simulink model "FOC_FPGA"  (R2020a)
settings: Solver=FixedStepDiscrete  StartTime=0.0  StopTime=1  FixedStep=2e-6  MaxStep=1e-4  RelTol=1e-3
values from neighbouring files (symbols this model uses):
  Ld = 0.008    [Thong_so_dong_co_FOC.m]
  Lq = 0.008    [Thong_so_dong_co_FOC.m]
  Omega = exp(-wc*Tp_SMO)    [Thong_so_dong_co_FOC.m]
  T_pulse = 5*10^(-5)    (= 5e-05)    [Thong_so_dong_co_FOC.m]
  Ts_idq = 1*10^(-4)    (= 0.0001)    [Thong_so_dong_co_FOC.m]
  Wc = exp(-500*Tp_SMO)    [Thong_so_dong_co_FOC.m]
  zp = 4    [Thong_so_dong_co_FOC.m]
undefined symbols (not defined in the file or in its folder): Inventor, PMSM
libraries: powerlib x11, modelsimlib x6, simulink x1
settings Model: Creator=ADMIN  LastModifiedBy=ADMIN
settings SolverCC: ZeroCrossAlgorithm=Adaptive
settings DebuggingCC: IgnoredZcDiagnostic=none

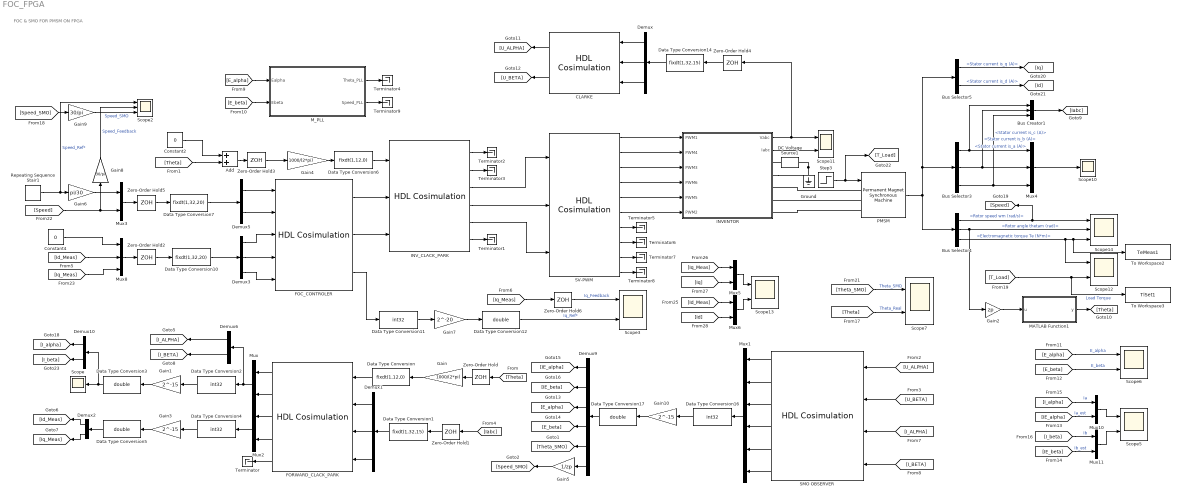
== system FOC_FPGA ==
  note: FOC & SMO FOR PMSM ON FPGA
  Add : Sum
  Bus Creator1 : BusCreator  Inputs=3
  Bus Selector3 : BusSelector  OutputSignals=Stator current is_a (A),Stator current is_b (A),Stator current is_c (A)
  Bus Selector4 : BusSelector  OutputSignals=Rotor speed wm (rad/s),Rotor angle thetam (rad),Electromagnetic torque Te (N*m)
  Bus Selector5 : BusSelector  OutputSignals=Stator current is_q (A),Stator current is_d (A)
  CLARKE : modelsimlib/HDL Cosimulation  PortPaths=/clarke/UA;/clarke/UB;/clarke/UC;/clarke/U_ALPHA;/clarke/U_BETA  PortModes=[1 1 1 2 2 ]  PortTimes=[-1,-1,-1,2e-6,2e-6]  PortSigns=[-1 -1 -1 -1 -1 ]  PortFracLengths=[0,0,0,0,0]  CommLocal=on  CommSharedMemory=on  CommPortNumber=4449  CommShowInfo=on  ClockPaths=/clarke/CLK  ClockModes=[2 ]  ClockTimes=[2e-8]  TclPreSimCommand="puts \"Running Simulink Cosimulation block.\""  TclPostSimCommand="puts \"done\""  TimingMode=s  TimingScaleFactor=1  idxCellArray={'UNUSED_VAR'}  CosimBypass=Full Simulation  AllowDirectFeedthrough=on  ProductName=EDA Simulator Link MQ  RunAutoTimescale=off  HdlClocks=0  PreRunTime=0  PreRunTimeUnit=ns
      settings: SourceProductBaseCode=ES
  Constant2 : Constant  Value=0
  Constant4 : Constant  Value=0
  DC Voltage Source1 : powerlib/Electrical Sources/DC Voltage Source  Amplitude=100  Measurements=None
  Data Type Conversion : DataTypeConversion  OutDataTypeStr=fixdt(1,12,0)
  Data Type Conversion1 : DataTypeConversion  OutDataTypeStr=fixdt(1,32,15)
  Data Type Conversion10 : DataTypeConversion  OutDataTypeStr=fixdt(1,32,20)
  Data Type Conversion{2,4,11,16} (4 alike) : DataTypeConversion  OutDataTypeStr=int32
  Data Type Conversion{3,5,12,17} (4 alike) : DataTypeConversion  OutDataTypeStr=double
  Data Type Conversion14 : DataTypeConversion  OutDataTypeStr=fixdt(1,32,15)
  Data Type Conversion6 : DataTypeConversion  OutDataTypeStr=fixdt(1,12,0)
  Data Type Conversion7 : DataTypeConversion  OutDataTypeStr=fixdt(1,32,20)
  Demux : Demux  Outputs=3
  Demux1 : Demux  Outputs=3
  Demux{2,5..6,10} (4 alike) : Demux  Outputs=2
  Demux3 : Demux  Outputs=3
  Demux9 : Demux  Outputs=6
  FOC_CONTROLER : modelsimlib/HDL Cosimulation  PortPaths=/foc_control/W_REF;/foc_control/W;/foc_control/I_DR;/foc_control/I_D;/foc_control/I_Q;/foc_control/U_D;/foc_control/U_Q;/foc_control/I_QR  PortModes=[1 1 1 1 1 2 2 2 ]  PortTimes=[-1,-1,-1,-1,-1,2e-6,2e-6,2e-6]  PortSigns=[-1 -1 -1 -1 -1 -1 -1 -1 ]  PortFracLengths=[0,0,0,0,0,0,0,0]  CommLocal=on  CommSharedMemory=on  CommPortNumber=4449  CommShowInfo=on  ClockPaths=/foc_control/CLK;/foc_control/CLK_200N  ClockModes=[2 2 ]  ClockTimes=[2e-8,2e-7]  TclPreSimCommand="puts \"Running Simulink Cosimulation block.\""  TclPostSimCommand="puts \"done\""  TimingMode=s  TimingScaleFactor=1  idxCellArray={'UNUSED_VAR'}  CosimBypass=Full Simulation  AllowDirectFeedthrough=on  ProductName=EDA Simulator Link MQ  RunAutoTimescale=off  HdlClocks=0  PreRunTime=0  PreRunTimeUnit=ns
      settings: SourceProductBaseCode=ES
  FORWARD_CLACK_PARK : modelsimlib/HDL Cosimulation  PortPaths=/forward_clack_park/ADDRESS;/forward_clack_park/IA;/forward_clack_park/IB;/forward_clack_park/IC;/forward_clack_park/I_ALPHA;/forward_clack_park/I_BETA;/forward_clack_park/I_D;/forward_clack_park/I_Q;/forward_clack_park/DONE  PortModes=[1 1 1 1 2 2 2 2 2 ]  PortTimes=[-1,-1,-1,-1,2e-6,2e-6,2e-6,2e-6,2e-6]  PortSigns=[-1 -1 -1 -1 -1 -1 -1 -1 -1 ]  PortFracLengths=[0,0,0,0,0,0,0,0,0]  CommLocal=on  CommSharedMemory=on  CommPortNumber=4449  CommShowInfo=on  ClockPaths=/forward_clack_park/CLK  ClockModes=[2 ]  ClockTimes=[2e-8]  TclPreSimCommand="puts \"Running Simulink Cosimulation block.\""  TclPostSimCommand="puts \"done\""  TimingMode=s  TimingScaleFactor=1  idxCellArray={'UNUSED_VAR'}  CosimBypass=Full Simulation  AllowDirectFeedthrough=on  ProductName=EDA Simulator Link MQ  RunAutoTimescale=off  HdlClocks=0  PreRunTime=0  PreRunTimeUnit=ns
      settings: SourceProductBaseCode=ES
  Gain : Gain  Gain=1000/(2*pi)
  Gain1 : Gain  Gain=2^-15
  Gain10 : Gain  Gain=2^-15
  Gain2 : Gain  Gain=zp
  Gain3 : Gain  Gain=2^-15
  Gain4 : Gain  Gain=1000/(2*pi)
  Gain5 : Gain  Gain=1/zp
  Gain6 : Gain  Gain=pi/30
  Gain7 : Gain  Gain=2^-20
  Gain8 : Gain  Gain=30/pi
  Gain9 : Gain  Gain=30/pi
  Ground : powerlib/Elements/Ground  LConnTagsString=a
  INVENTOR : Subsystem  AncestorBlock=PMSM/Inventor
  INV_CLACK_PARK : modelsimlib/HDL Cosimulation  PortPaths=/inverse_clack_park/ADDRESS;/inverse_clack_park/U_D;/inverse_clack_park/U_Q;/inverse_clack_park/U_ALPHA;/inverse_clack_park/U_BETA;/inverse_clack_park/VREFA;/inverse_clack_park/VREFB;/inverse_clack_park/VREFC;/inverse_clack_park/DONE  PortModes=[1 1 1 2 2 2 2 2 2 ]  PortTimes=[-1,-1,-1,2e-6,2e-6,2e-6,2e-6,2e-6,2e-6]  PortSigns=[-1 -1 -1 -1 -1 -1 -1 -1 -1 ]  PortFracLengths=[0,0,0,0,0,0,0,0,0]  CommLocal=on  CommSharedMemory=on  CommPortNumber=4449  CommShowInfo=on  ClockPaths=/inverse_clack_park/CLK  ClockModes=[2 ]  ClockTimes=[2e-8]  TclPreSimCommand="puts \"Running Simulink Cosimulation block.\""  TclPostSimCommand="puts \"done\""  TimingMode=s  TimingScaleFactor=1  idxCellArray={'UNUSED_VAR'}  CosimBypass=Full Simulation  AllowDirectFeedthrough=on  ProductName=EDA Simulator Link MQ  RunAutoTimescale=off  HdlClocks=0  PreRunTime=0  PreRunTimeUnit=ns
      settings: SourceProductBaseCode=ES
  MATLAB Function1 : MATLAB Function  TreatAsAtomicUnit=on
  M_PLL : Subsystem
  Mux{,2..3,5..6,10..11} (7 alike) : Mux  Inputs=2
  Mux1 : Mux  Inputs=6
  Mux4 : Mux  Inputs=3
  Mux8 : Mux  Inputs=3
  PMSM : powerlib/Machines/Permanent Magnet Synchronous Machine  NbPhases=3  FluxDistribution=Sinusoidal  RotorType=Salient-pole  MechanicalLoad=Torque Tm  PresetModel=No  ShowDetailedParameters=on  MeasurementBus=off  Resistance=3.2  Inductance=8.5e-3  dqInductances=[Ld Lq]  La=0.008  MachineConstant=Flux linkage established by magnets (V.s)  Flux=0.0471405  VoltageCst=34.2014  TorqueCst=0.28284  Flat=120  Mechanical=[1.4e-05 4.5e-06 4]  PolePairs=2  InitialConditions=[0,0, 0,0]  InitialConditions5ph=[0 0 0 0 0 0]  RefAngle=Aligned with phase A axis (original Park)  IterativeDiscreteModel=Trapezoidal non iterative  TsBlock=-1  TsPowergui=0
  Repeating Sequence Stair1 : simulink/Sources/Repeating Sequence Stair  OutValues=[300 600 900 -600 -300 ].'  tsamp=0.2  OutMin=[]  OutMax=[]  OutDataTypeStr=double  OutputDataTypeScalingMode=double  OutDataType=fixdt(0,8)  ConRadixGroup=Best Precision: Vector-wise  OutScaling=2^-12
  SMO OBSERVER : modelsimlib/HDL Cosimulation  PortPaths=/smo_observer/U_ALPHA;/smo_observer/U_BETA;/smo_observer/I_ALPHA;/smo_observer/I_BETA;/smo_observer/IE_ALPHA;/smo_observer/IE_BETA;/smo_observer/E_ALPHA;/smo_observer/E_BETA;/smo_observer/THETA;/smo_observer/SPEED  PortModes=[1 1 1 1 2 2 2 2 2 2 ]  PortTimes=[-1,-1,-1,-1,2e-6,2e-6,2e-6,2e-6,2e-6,2e-6]  PortSigns=[-1 -1 -1 -1 -1 -1 -1 -1 -1 -1 ]  PortFracLengths=[0,0,0,0,0,0,0,0,0,0]  CommLocal=on  CommSharedMemory=on  CommPortNumber=4449  CommShowInfo=on  ClockPaths=/smo_observer/CLK;/smo_observer/CLK_80N  ClockModes=[2 2 ]  ClockTimes=[2e-8,8e-8]  TclPreSimCommand="puts \"Running Simulink Cosimulation block.\""  TclPostSimCommand="puts \"done\""  TimingMode=s  TimingScaleFactor=1  idxCellArray={'UNUSED_VAR'}  CosimBypass=Full Simulation  AllowDirectFeedthrough=on  ProductName=EDA Simulator Link MQ  RunAutoTimescale=off  HdlClocks=0  PreRunTime=0  PreRunTimeUnit=ns
      settings: SourceProductBaseCode=ES
  SV-PWM : modelsimlib/HDL Cosimulation  PortPaths=/svpwm/VREF1;/svpwm/VREF2;/svpwm/VREF3;/svpwm/PWM1;/svpwm/PWM2;/svpwm/PWM3;/svpwm/PWM4;/svpwm/PWM5;/svpwm/PWM6;/svpwm/CMPR1;/svpwm/CMPR2;/svpwm/CMPR3;/svpwm/Q  PortModes=[1 1 1 2 2 2 2 2 2 2 2 2 2 ]  PortTimes=[-1,-1,-1,2e-6,2e-6,2e-6,2e-6,2e-6,2e-6,1,1,1,1]  PortSigns=[-1 -1 -1 -1 -1 -1 -1 -1 -1 -1 -1 -1 -1 ]  PortFracLengths=[0,0,0,0,0,0,0,0,0,0,0,0,0]  CommLocal=on  CommSharedMemory=on  CommPortNumber=4449  CommShowInfo=on  ClockPaths=/svpwm/CLK;/svpwm/CLK_200N  ClockModes=[2 2 ]  ClockTimes=[2e-8,2e-7]  TclPreSimCommand="puts \"Running Simulink Cosimulation block.\""  TclPostSimCommand="puts \"done\""  TimingMode=s  TimingScaleFactor=1  idxCellArray={'UNUSED_VAR'}  CosimBypass=Full Simulation  AllowDirectFeedthrough=on  ProductName=EDA Simulator Link MQ  RunAutoTimescale=off  HdlClocks=0  PreRunTime=0  PreRunTimeUnit=ns
      settings: SourceProductBaseCode=ES
  Scope : Scope
  Scope10 : Scope
  Scope{3,5..7,11..13} (7 alike) : Scope  NumInputPorts=2
  Scope14 : Scope  NumInputPorts=3
  Scope2 : Scope  NumInputPorts=3
  Step3 : Step  Time=0.15  Before=0.2  After=0.3  SampleTime=0
  Terminator{,1..9} (10 alike) : Terminator
  To Workspace2 : ToWorkspace  VariableName=TeMeas1  SampleTime=-1
  To Workspace3 : ToWorkspace  VariableName=TlSet1  SampleTime=-1
  Zero-Order Hold{,1..5} (6 alike) : ZeroOrderHold  SampleTime=2e-6
  Zero-Order Hold6 : ZeroOrderHold  SampleTime=Ts_idq
  wires:
  [Iq] -> Mux5/2
  Bus Creator1/1 -> [Iabc]
  [T_Load] -> To Workspace3/1, Scope12/2  "Load Torque"
  Mux6/1 -> Scope13/2
  Bus Selector3/1 -> Bus Creator1/1, Mux4/1  "<Stator current is_a (A)>"
  [Iq_Meas] -> Mux5/1
  INVENTOR/2("Iabc ") -> Scope11/2
  Mux4/1 -> Scope10/1
  PMSM/1 -> Bus Selector4/1, Bus Selector5/1, Bus Selector3/1
  Bus Selector3/3 -> Bus Creator1/3, Mux4/3  "<Stator current is_c (A)>"
  [Id] -> Mux6/2
  Mux5/1 -> Scope13/1
  Bus Selector4/1 -> Scope14/1, [Speed]  "<Rotor speed wm (rad/s)>"
  Step3/1 -> PMSM/1, [T_Load]
  Bus Selector5/1 -> [Iq]  "<Stator current is_q (A)>"
  MATLAB Function1/1(y) -> [Theta]
  Bus Selector4/2 -> Scope14/2, Gain2/1  "<Rotor angle thetam (rad)>"
  Gain2/1 -> MATLAB Function1/1(u)
  [Id_Meas] -> Mux6/1
  Bus Selector3/2 -> Bus Creator1/2, Mux4/2  "<Stator current is_b (A)>"
  Bus Selector4/3 -> Scope12/1, To Workspace2/1, Scope14/3  "<Electromagnetic torque Te (N*m)>"
  Bus Selector5/2 -> [Id]  "<Stator current is_d (A)>"
  [Theta] -> Zero-Order Hold/1
  Zero-Order Hold/1 -> Gain/1
  Gain/1 -> Data Type Conversion/1
  Data Type Conversion/1 -> FORWARD_CLACK_PARK/1
  Demux1/3 -> FORWARD_CLACK_PARK/4
  Demux1/2 -> FORWARD_CLACK_PARK/3
  Demux1/1 -> FORWARD_CLACK_PARK/2
  Data Type Conversion1/1 -> Demux1/1
  Zero-Order Hold1/1 -> Data Type Conversion1/1
  [Iabc] -> Zero-Order Hold1/1
  FORWARD_CLACK_PARK/1 -> Mux/1
  FORWARD_CLACK_PARK/2 -> Mux/2
  Mux/1 -> Demux6/1, Data Type Conversion2/1
  Data Type Conversion2/1 -> Gain1/1
  Gain1/1 -> Data Type Conversion3/1
  Data Type Conversion3/1 -> Scope/1, Demux10/1
  Gain3/1 -> Data Type Conversion5/1
  Data Type Conversion4/1 -> Gain3/1
  Mux2/1 -> Data Type Conversion4/1
  FORWARD_CLACK_PARK/4 -> Mux2/2
  FORWARD_CLACK_PARK/3 -> Mux2/1
  Data Type Conversion5/1 -> Demux2/1
  Demux2/1 -> [Id_Meas]
  Demux2/2 -> [Iq_Meas]
  Data Type Conversion6/1 -> INV_CLACK_PARK/1
  Gain4/1 -> Data Type Conversion6/1
  Zero-Order Hold3/1 -> Gain4/1
  Add/1 -> Zero-Order Hold3/1
  [Theta] -> Add/2
  Constant2/1 -> Add/1
  Repeating Sequence Stair1/1 -> Gain6/1, Scope2/1  "Speed_Ref*"
  Mux8/1 -> Zero-Order Hold2/1
  Data Type Conversion10/1 -> Demux3/1
  FOC_CONTROLER/1 -> INV_CLACK_PARK/2
  FOC_CONTROLER/2 -> INV_CLACK_PARK/3
  [Speed] -> Gain8/1, Mux3/2
  Demux3/2 -> FOC_CONTROLER/4
  Demux3/3 -> FOC_CONTROLER/5
  Demux3/1 -> FOC_CONTROLER/3
  Constant4/1 -> Mux8/1
  Zero-Order Hold2/1 -> Data Type Conversion10/1
  [Id_Meas] -> Mux8/2
  [Iq_Meas] -> Mux8/3
  Zero-Order Hold5/1 -> Data Type Conversion7/1
  Data Type Conversion7/1 -> Demux5/1
  Demux5/1 -> FOC_CONTROLER/1
  Demux5/2 -> FOC_CONTROLER/2
  Mux3/1 -> Zero-Order Hold5/1
  Gain6/1 -> Mux3/1
  Data Type Conversion11/1 -> Gain7/1
  Gain7/1 -> Data Type Conversion12/1
  FOC_CONTROLER/3 -> Data Type Conversion11/1
  [Iq_Meas] -> Zero-Order Hold6/1
  FORWARD_CLACK_PARK/5 -> Terminator/1
  INV_CLACK_PARK/6 -> Terminator1/1
  INV_CLACK_PARK/5 -> SV-PWM/3
  SV-PWM/7 -> Terminator5/1
  SV-PWM/8 -> Terminator6/1
  SV-PWM/9 -> Terminator7/1
  SV-PWM/10 -> Terminator8/1
  INV_CLACK_PARK/3 -> SV-PWM/1
  SV-PWM/1 -> INVENTOR/1("PWM1 ")
  SV-PWM/2 -> INVENTOR/2("PWM4 ")
  SV-PWM/3 -> INVENTOR/3("PWM3 ")
  SV-PWM/4 -> INVENTOR/4("PWM6 ")
  SV-PWM/5 -> INVENTOR/5("PWM5 ")
  SV-PWM/6 -> INVENTOR/6("PWM2 ")
  Gain8/1 -> Scope2/2  "Speed_Feedback"
  Demux6/1 -> [I_ALPHA]
  Demux6/2 -> [I_BETA]
  Data Type Conversion17/1 -> Demux9/1
  Mux1/1 -> Data Type Conversion16/1
  Data Type Conversion16/1 -> Gain10/1
  Gain10/1 -> Data Type Conversion17/1
  Mux10/1 -> Scope5/1
  Mux11/1 -> Scope5/2
  [IE_alpha] -> Mux10/2  "Ia_est"
  [IE_beta] -> Mux11/2  "Ib_est"
  [I_beta] -> Mux11/1  "Ib"
  [I_alpha] -> Mux10/1  "Ia"
  [E_beta] -> Scope6/2  "E_beta"
  [E_alpha] -> Scope6/1  "E_alpha"
  Demux10/1 -> [I_alpha]
  Demux10/2 -> [I_beta]
  INVENTOR/1("Vabc ") -> Scope11/1, Zero-Order Hold4/1
  Data Type Conversion12/1 -> Scope3/2  "Iq_Ref*"
  Zero-Order Hold6/1 -> Scope3/1  "Iq_Feedback"
  INV_CLACK_PARK/4 -> SV-PWM/2
  Demux/3 -> CLARKE/3
  Demux/2 -> CLARKE/2
  Demux/1 -> CLARKE/1
  [Speed_SMO] -> Gain9/1
  Gain9/1 -> Scope2/3  "Speed_SMO"
  Zero-Order Hold4/1 -> Data Type Conversion14/1
  Data Type Conversion14/1 -> Demux/1
  CLARKE/1 -> [U_ALPHA]
  CLARKE/2 -> [U_BETA]
  [E_alpha] -> M_PLL/1(Ealpha)
  [E_beta] -> M_PLL/2(Ebeta)
  [I_ALPHA] -> SMO OBSERVER/3
  [I_BETA] -> SMO OBSERVER/4
  [U_BETA] -> SMO OBSERVER/2
  [U_ALPHA] -> SMO OBSERVER/1
  SMO OBSERVER/1 -> Mux1/1
  SMO OBSERVER/4 -> Mux1/4
  SMO OBSERVER/5 -> Mux1/5
  SMO OBSERVER/3 -> Mux1/3
  SMO OBSERVER/2 -> Mux1/2
  Demux9/1 -> [IE_alpha]
  Demux9/2 -> [IE_beta]
  Demux9/3 -> [E_alpha]
  Demux9/4 -> [E_beta]
  Demux9/5 -> [Theta_SMO]
  INV_CLACK_PARK/2 -> Terminator3/1
  INV_CLACK_PARK/1 -> Terminator2/1
  SMO OBSERVER/6 -> Mux1/6
  Demux9/6 -> Gain5/1
  [Theta_SMO] -> Scope7/1  "Theta_SMO"
  [Theta] -> Scope7/2  "Theta_Real"
  M_PLL/2(Speed_PLL) -> Terminator9/1
  M_PLL/1(Theta_PLL) -> Terminator4/1
  Gain5/1 -> [Speed_SMO]
  connections:
  INVENTOR/RConn2 -- Ground/LConn1 -- DC Voltage Source1/LConn1
  DC Voltage Source1/RConn1 -- INVENTOR/RConn1
  PMSM/LConn1 -- INVENTOR/RConn3
  PMSM/LConn2 -- INVENTOR/RConn4
  PMSM/LConn3 -- INVENTOR/RConn5

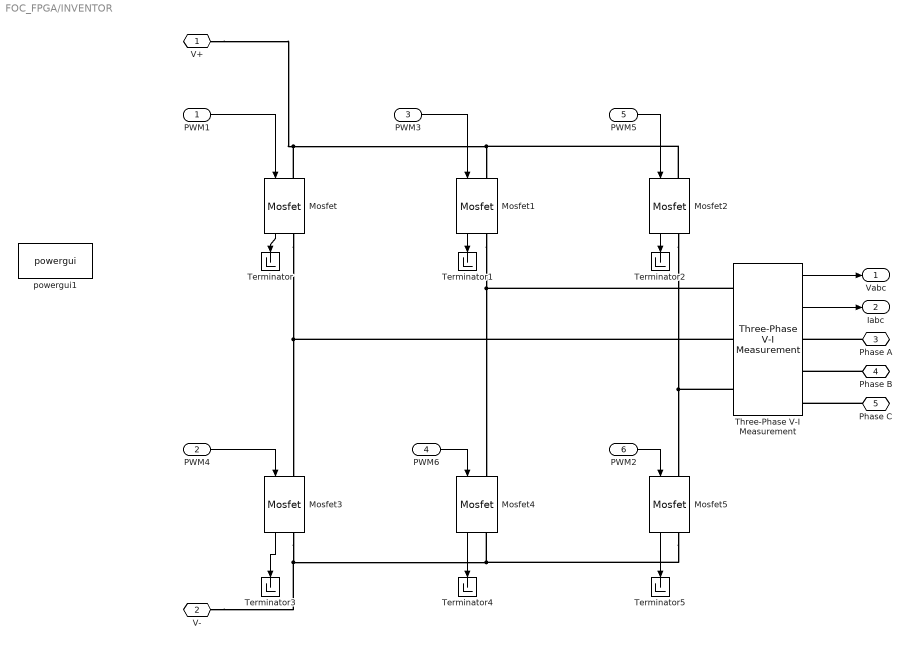
== system FOC_FPGA/INVENTOR ==
  "PWM1 " : Inport
  "PWM4 " : Inport  Port=2
  "PWM3 " : Inport  Port=3
  "PWM6 " : Inport  Port=4
  "PWM5 " : Inport  Port=5
  "PWM2 " : Inport  Port=6
  Mosfet{,1..5} (6 alike) : powerlib/Power Electronics/Mosfet  Ron=0.1  Lon=0  Rd=0.01  Vfd=0  IC=0  Rs=1e5  Cs=inf  Measurements=on
  Terminator{,1..5} (6 alike) : Terminator
  Three-Phase V-I Measurement : powerlib/Measurements/Three-Phase V-I Measurement  VoltageMeasurement=phase-to-phase  SetLabelV=off  LabelV=Vabc  Vpu=off  VpuLL=off  CurrentMeasurement=yes  SetLabelI=off  LabelI=Iabc  Ipu=off  Pbase=100e6  Vbase=500e3  OutputType=Complex  PhasorSimulation=off  PSBequivalent=0
  powergui1 : powerlib/powergui  Priority=1  SimulationMode=Discrete  SampleTime=2e-6  frequency=60  Iterations=50  frequencyindice=0  Pbase=100e6  ErrMax=1e-4  UnitsV=kV  UnitsW=MW  buscounter=0  FunctionMessages=off  echomessages=off  EnableUseOfTLC=off  CurrentSourceSwitches=off  DisableSnubberDevices=off  DisableRonSwitches=off  DisableVfSwitches=off  DisplayEquations=off  AutomaticDiscreteSolvers=off  SolverType=Tustin/Backward Euler (TBE)  Interpol=off  ExternalGateDelay=off  methode=off  Ts=100  x0status=blocks  SPID=on  SwTol=0  HookPort=off  NonlinearTolerance=1e-4  nMaxIteration=100  ContinueOnMaxIteration=off  RestoreLinks=warning  ResistiveCurrentMeasurement=off  Frange=[0:2:500]  Ylog=off  Xlog=on  ShowGrid=off  save=off  variable=ZData  structure=0  ZoomFFT=off  StartTime=0.0  cycles=1  DisplayStyle=1  fundamental=60  FreqAxis=off  MaxFrequency=1000  frequencyindicesteady=1  RmsSteady=1  display=off
  "V+ " : PMIOPort  Side=Right
  "V- " : PMIOPort  Port=2  Side=Right
  "Phase A " : PMIOPort  Port=3  Side=Right
  "Phase B " : PMIOPort  Port=4  Side=Right
  Phase C : PMIOPort  Port=5  Side=Right
  "Vabc " : Outport  VectorParamsAs1DForOutWhenUnconnected=off
  "Iabc " : Outport  Port=2  VectorParamsAs1DForOutWhenUnconnected=off
  wires:
  Mosfet5/1 -> Terminator5/1
  Mosfet4/1 -> Terminator4/1
  Mosfet3/1 -> Terminator3/1
  Mosfet2/1 -> Terminator2/1
  Mosfet1/1 -> Terminator1/1
  Mosfet/1 -> Terminator/1
  Three-Phase V-I Measurement/2 -> "Iabc "/1
  Three-Phase V-I Measurement/1 -> "Vabc "/1
  "PWM4 "/1 -> Mosfet3/1
  "PWM1 "/1 -> Mosfet/1
  "PWM5 "/1 -> Mosfet2/1
  "PWM2 "/1 -> Mosfet5/1
  "PWM6 "/1 -> Mosfet4/1
  "PWM3 "/1 -> Mosfet1/1
  connections:
  Phase C/RConn1 -- Three-Phase V-I Measurement/RConn3
  "Phase B "/RConn1 -- Three-Phase V-I Measurement/RConn2
  "Phase A "/RConn1 -- Three-Phase V-I Measurement/RConn1
  "V- "/RConn1 -- Mosfet3/RConn1 -- Mosfet4/RConn1 -- Mosfet5/RConn1
  "V+ "/RConn1 -- Mosfet/LConn1 -- Mosfet1/LConn1 -- Mosfet2/LConn1
  Mosfet2/RConn1 -- Three-Phase V-I Measurement/LConn3 -- Mosfet5/LConn1
  Mosfet1/RConn1 -- Three-Phase V-I Measurement/LConn1 -- Mosfet4/LConn1
  Mosfet/RConn1 -- Three-Phase V-I Measurement/LConn2 -- Mosfet3/LConn1

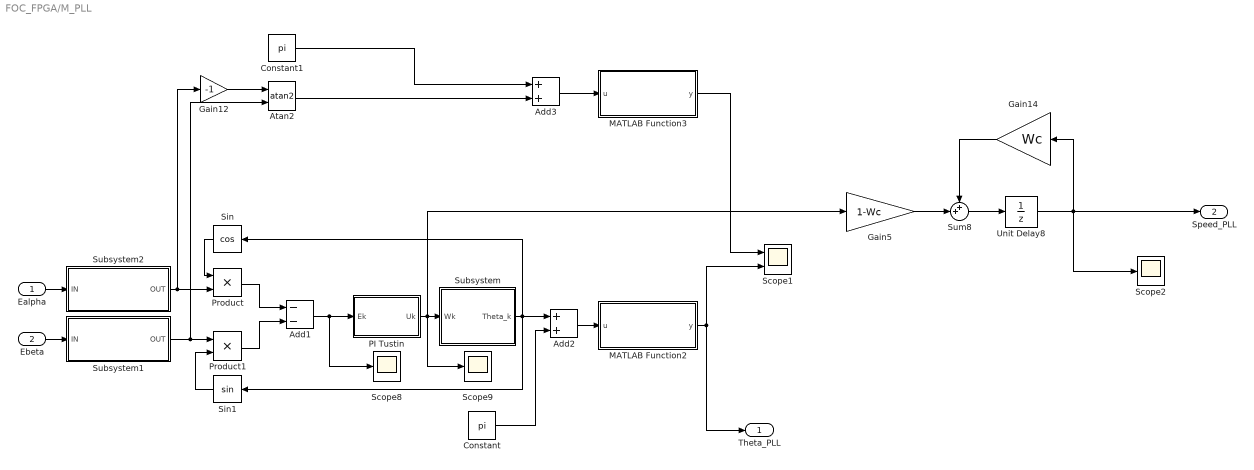
== system FOC_FPGA/M_PLL ==
  Ealpha : Inport
  Ebeta : Inport  Port=2
  Add1 : Sum  Inputs=--
  Add2 : Sum
  Add3 : Sum
  Atan2 : Trigonometry  Operator=atan2
  Constant : Constant  Value=pi
  Constant1 : Constant  Value=pi
  Gain12 : Gain  Gain=-1
  Gain14 : Gain  Gain=Wc
  Gain5 : Gain  Gain=1-Wc
  MATLAB Function2 : MATLAB Function  TreatAsAtomicUnit=on
  MATLAB Function3 : MATLAB Function  TreatAsAtomicUnit=on
  PI Tustin : Subsystem
  Product : Product
  Product1 : Product
  Scope1 : Scope  NumInputPorts=2
  Scope2 : Scope
  Scope8 : Scope
  Scope9 : Scope
  Sin : Trigonometry  Operator=cos
  Sin1 : Trigonometry
  Subsystem : Subsystem
  Subsystem1 : Subsystem
  Subsystem2 : Subsystem
  Sum8 : Sum  Inputs=++|
  Unit Delay8 : UnitDelay  InitialCondition=0.1  SampleTime=T_pulse  HasFrameUpgradeWarning=on
  Theta_PLL : Outport
  Speed_PLL : Outport  Port=2
  wires:
  Gain5/1 -> Sum8/2
  Gain14/1 -> Sum8/1
  Sin/1 -> Product/1
  Subsystem2/1(OUT) -> Gain12/1, Product/2
  Sin1/1 -> Product1/2
  Ebeta/1 -> Subsystem1/1(IN)
  Add1/1 -> Scope8/1, PI Tustin/1(Ek)
  PI Tustin/1(Uk) -> Scope9/1, Gain5/1, Subsystem/1(Wk)
  Sum8/1 -> Unit Delay8/1
  MATLAB Function2/1(y) -> Theta_PLL/1, Scope1/2
  Atan2/1 -> Add3/2
  Product/1 -> Add1/1
  Unit Delay8/1 -> Scope2/1, Speed_PLL/1, Gain14/1
  Subsystem/1(Theta_k) -> Add2/1, Sin/1, Sin1/1
  Add2/1 -> MATLAB Function2/1(u)
  Add3/1 -> MATLAB Function3/1(u)
  Product1/1 -> Add1/2
  Ealpha/1 -> Subsystem2/1(IN)
  Subsystem1/1(OUT) -> Atan2/2, Product1/1
  Constant/1 -> Add2/2
  Gain12/1 -> Atan2/1
  MATLAB Function3/1(y) -> Scope1/1
  Constant1/1 -> Add3/1

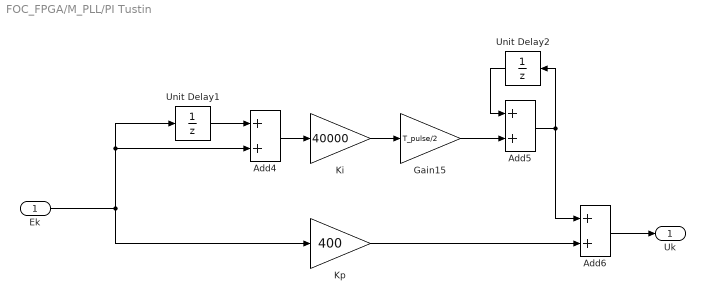
== system FOC_FPGA/M_PLL/PI Tustin ==
  Ek : Inport
  Add4 : Sum
  Add5 : Sum
  Add6 : Sum
  Gain15 : Gain  Gain=T_pulse/2
  Ki : Gain  Gain=40000
  Kp : Gain  Gain=400
  Unit Delay1 : UnitDelay  SampleTime=T_pulse  HasFrameUpgradeWarning=on
  Unit Delay2 : UnitDelay  SampleTime=T_pulse  HasFrameUpgradeWarning=on
  Uk : Outport
  wires:
  Kp/1 -> Add6/2
  Gain15/1 -> Add5/2
  Ki/1 -> Gain15/1
  Add5/1 -> Unit Delay2/1, Add6/1
  Add4/1 -> Ki/1
  Ek/1 -> Kp/1, Add4/2, Unit Delay1/1
  Unit Delay2/1 -> Add5/1
  Unit Delay1/1 -> Add4/1
  Add6/1 -> Uk/1

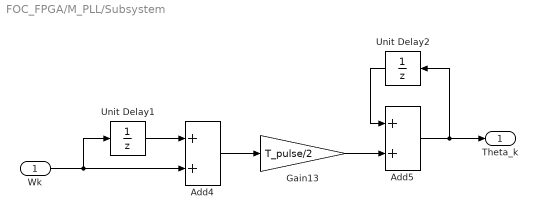
== system FOC_FPGA/M_PLL/Subsystem ==
  Wk : Inport
  Add4 : Sum
  Add5 : Sum
  Gain13 : Gain  Gain=T_pulse/2
  Unit Delay1 : UnitDelay  SampleTime=T_pulse  HasFrameUpgradeWarning=on
  Unit Delay2 : UnitDelay  InitialCondition=pi  SampleTime=T_pulse  HasFrameUpgradeWarning=on
  Theta_k : Outport
  wires:
  Wk/1 -> Unit Delay1/1, Add4/2
  Gain13/1 -> Add5/2
  Add4/1 -> Gain13/1
  Add5/1 -> Theta_k/1, Unit Delay2/1
  Unit Delay1/1 -> Add4/1
  Unit Delay2/1 -> Add5/1

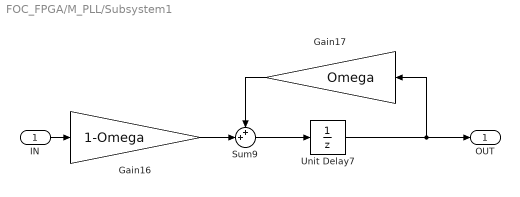
== system FOC_FPGA/M_PLL/Subsystem1 ==
  IN : Inport
  Gain16 : Gain  Gain=1-Omega
  Gain17 : Gain  Gain=Omega
  Sum9 : Sum  Inputs=++|
  Unit Delay7 : UnitDelay  SampleTime=T_pulse  HasFrameUpgradeWarning=on
  OUT : Outport
  wires:
  Gain17/1 -> Sum9/1
  Unit Delay7/1 -> Gain17/1, OUT/1
  Sum9/1 -> Unit Delay7/1
  Gain16/1 -> Sum9/2
  IN/1 -> Gain16/1

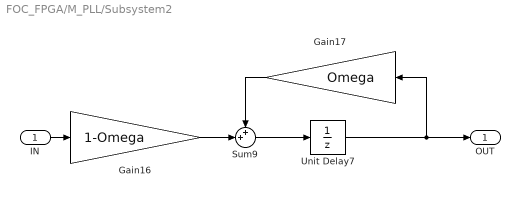
== system FOC_FPGA/M_PLL/Subsystem2 ==
  IN : Inport
  Gain16 : Gain  Gain=1-Omega
  Gain17 : Gain  Gain=Omega
  Sum9 : Sum  Inputs=++|
  Unit Delay7 : UnitDelay  SampleTime=T_pulse  HasFrameUpgradeWarning=on
  OUT : Outport
  wires:
  Gain17/1 -> Sum9/1
  Unit Delay7/1 -> Gain17/1, OUT/1
  Sum9/1 -> Unit Delay7/1
  Gain16/1 -> Sum9/2
  IN/1 -> Gain16/1

== matlab function FOC_FPGA/MATLAB Function1 ==
  data: u input; y output
function y = Adjust_Angle(u)
temp = u ;
temp1 = mod(temp,2*pi);
if temp1 < 0
    temp1 = temp1 + 2*pi;
else 
    temp1 = temp1 ;
end
y =   temp1 ;

== matlab function FOC_FPGA/M_PLL/MATLAB Function2 ==
  settings: updateMethod=DISCRETE  sampleTime=T_pulse
  data: u input; y output
function y = Adjust_Angle(u)
temp = u ;
temp1 = mod(temp,2*pi);
if temp1 < 0
    temp1 = temp1 + 2*pi;
else 
    temp1 = temp1 ;
end
y =   temp1 ;

== matlab function FOC_FPGA/M_PLL/MATLAB Function3 ==
  settings: updateMethod=DISCRETE  sampleTime=T_pulse
  data: u input; y output
function y = Adjust_Angle(u)
temp = u ;
temp1 = mod(temp,2*pi);
if temp1 < 0
    temp1 = temp1 + 2*pi;
else 
    temp1 = temp1 ;
end
y =   temp1 ;
